simulink model "rle9"  (R2025b)
settings: Solver=FixedStepAuto  StartTime=0.0  StopTime=t_stop  FixedStep=1e-3  MaxStep=1e-3  RelTol=1e-3
values from neighbouring files (symbols this model uses):
  Kp = 1    [rlelog9_.m]
  R = 0.725    [rlelog9_.m]
undefined symbols (not defined in the file or in its folder): den_ac, num_ac
settings Model: Creator=t0900  LastModifiedBy=t0900

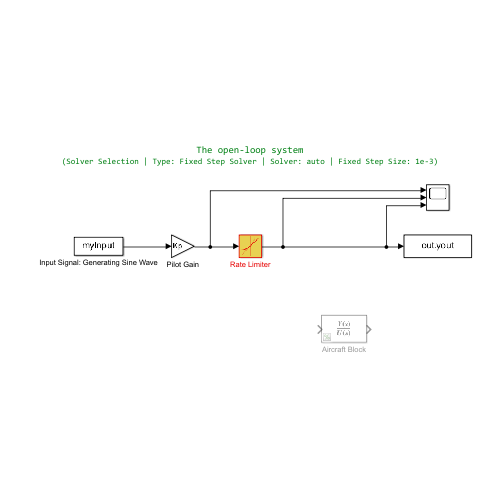
[thumbnail: Simulink's stored preview of the top-level diagram]
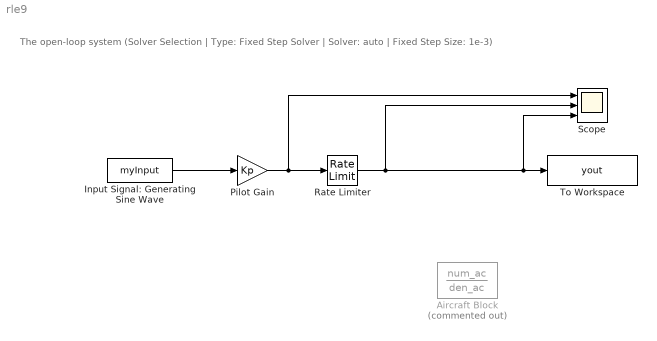
== system rle9 ==
  note: The open-loop system
      | (Solver Selection | Type: Fixed Step Solver | Solver: auto | Fixed Step Size: 1e-3)
  Aircraft Block : TransferFcn  Commented=on  Numerator=num_ac  Denominator=den_ac
  Input Signal: Generating Sine Wave : FromWorkspace  VariableName=myInput
  Pilot Gain : Gain  Gain=Kp
  Rate Limiter : RateLimiter  RisingSlewLimit=R  FallingSlewLimit=-R
  Scope : Scope  NumInputPorts=3
      settings: ActiveDisplayYMinimum=-4.3749954725549358  ActiveDisplayYMaximum=4.3749951589791722
  To Workspace : ToWorkspace  VariableName=yout  SampleTime=-1
  wires:
  Input Signal: Generating Sine Wave/1 -> Pilot Gain/1
  Pilot Gain/1 -> Scope/1, Rate Limiter/1
  Rate Limiter/1 -> Scope/3, To Workspace/1, Scope/2
